simulink model "ship_induction_motor_propulsion_extended_linear"  (R2016b)
settings: Solver=VariableStepAuto  StartTime=0.0  StopTime=500  FixedStep=1e-6
values from neighbouring files (symbols this model uses):
  a = -5.4036    [lin_propulsion_params.m]    (also in robust_lin_propulsion_params_zs.m; ship_induction_motor_propulsion_extended_linear.m)
  b = -3.499    [lin_propulsion_params.m]    (also in robust_lin_propulsion_params_zs.m; ship_induction_motor_propulsion_extended_linear.m)
  J_ind = 4.1    [linear_motor_params.m]    (also in robust_linear_motor_params.m = ureal('J_ind',4.1,'Percentage',range); ship_induction_motor_propulsion_extended_linear.m)
  L_ad_ind = L_aq_ind    (= 0.00307086614173)    [linear_motor_params.m]    (also in robust_linear_motor_params.m = L_aq_ind; ship_induction_motor_propulsion_extended_linear.m)
  L_aq_ind = 1/(1/L_M_ind + 1/L_ls_ind + 1/L_lr_ind)    (= 0.00307086614173)    [linear_motor_params.m]    (also in robust_linear_motor_params.m = 1/(1/L_M_ind + 1/L_ls_ind + 1/L_lr_ind); ship_induction_motor_propulsion_extended_linear.m)
  L_eq = L_ls_ind + L_M_ind *(L_lr_ind)/(L_lr_ind+L_M_ind)    (= 0.0188613861386)    [linear_motor_params.m]    (also in robust_linear_motor_params.m = L_ls_ind + L_M_ind *(L_lr_ind)/(L_lr_ind+L_M_ind); ship_induction_motor_propulsion_extended_linear.m)
  L_lr_ind = 15e-3    (= 0.015)    [linear_motor_params.m]    (also in robust_linear_motor_params.m = ureal('L_lr_ind',15e-3, 'Percentage',range); ship_induction_motor_propulsion_extended_linear.m)
  L_ls_ind = 15e-3    (= 0.015)    [linear_motor_params.m]    (also in robust_linear_motor_params.m = ureal('L_ls_ind',15e-3, 'Percentage',range); ship_induction_motor_propulsion_extended_linear.m)
  L_M_ind = 5.2e-3    (= 0.0052)    [linear_motor_params.m]    (also in robust_linear_motor_params.m = ureal('L_M_ind',5.2e-3, 'Percentage',range); ship_induction_motor_propulsion_extended_linear.m)
  p = 6.58    [lin_propulsion_params.m]    (also in robust_lin_propulsion_params_zs.m; ship_induction_motor_propulsion_extended_linear.m)
  P_ind = 4    [linear_motor_params.m]    (also in robust_linear_motor_params.m; ship_induction_motor_propulsion_extended_linear.m)
  q = 5.0245    [lin_propulsion_params.m]    (also in robust_lin_propulsion_params_zs.m; ship_induction_motor_propulsion_extended_linear.m)
  r_r_ind = 4.6e-3    (= 0.0046)    [linear_motor_params.m]    (also in robust_linear_motor_params.m = ureal('r_r_ind', 4.6e-3, 'Percentage', range); ship_induction_motor_propulsion_extended_linear.m)
  r_s_ind = 7.6e-3    (= 0.0076)    [linear_motor_params.m]    (also in robust_linear_motor_params.m = ureal('r_s_ind', 7.6e-3, 'Percentage', range); ship_induction_motor_propulsion_extended_linear.m)
  T_r_ind = L_lr_ind/r_r_ind    (= 3.26086956522)    [linear_motor_params.m]    (also in robust_linear_motor_params.m = L_lr_ind/r_r_ind; ship_induction_motor_propulsion_extended_linear.m)
  T_s_est = 1e-2    (= 0.01)    [linear_motor_params.m]    (also in robust_linear_motor_params.m; ship_induction_motor_propulsion_extended_linear.m)
  Tn = 7.83    [lin_propulsion_params.m]    (also in robust_lin_propulsion_params_zs.m; ship_induction_motor_propulsion_extended_linear.m)
  Ts = 1e-3    (= 0.001)    [linear_motor_params.m]    (also in robust_linear_motor_params.m; ship_induction_motor_propulsion_extended_linear.m)
  Tth = 2    [lin_propulsion_params.m]    (also in robust_lin_propulsion_params_zs.m; ship_induction_motor_propulsion_extended_linear.m)
  Tv = 115.69    [lin_propulsion_params.m]    (also in robust_lin_propulsion_params_zs.m; ship_induction_motor_propulsion_extended_linear.m)
libraries: simulink x10
settings Model: Creator=z003vh9b  LastModifiedBy=z003vh9b

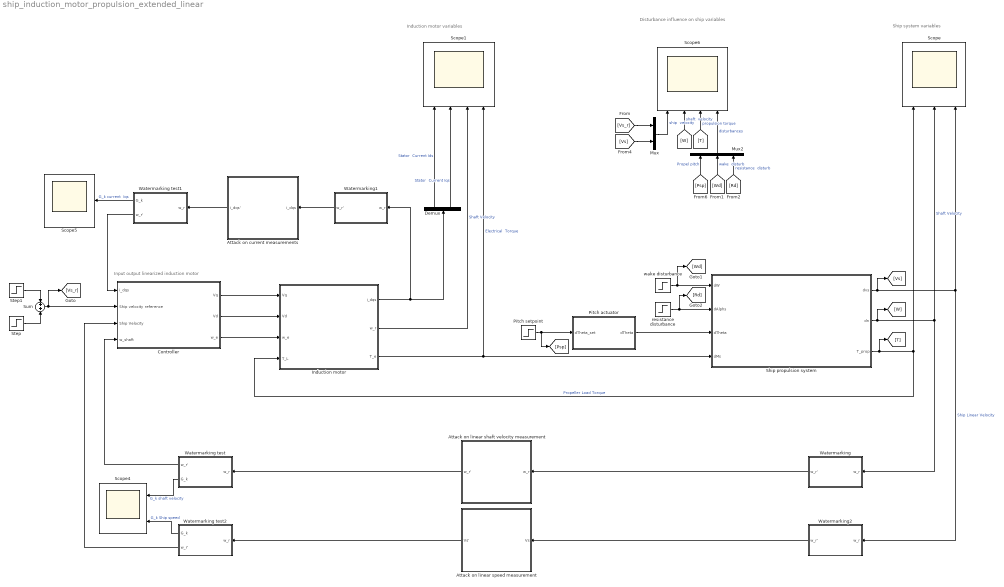
== system ship_induction_motor_propulsion_extended_linear ==
  note: Input output linearized induction motor
  note: Induction motor variables
  note: Ship system variables
  note: Disturbance influence on
      | ship variables
  Attack on current measurements : Subsystem
  Attack on linear shaft velocity measurement : Subsystem
  Attack on linear speed measurement : Subsystem
  Controller : Subsystem
  Demux : Demux  Outputs=2
  Induction motor : Subsystem  mask{N=10e-3, Fs_n=1e3}
      mask prompts: N "Current Noise magnitude"; Fs_n "Current Noise frequency"
  Mux : Mux  Inputs=2
  Mux2 : Mux  Inputs=3
  Pitch actuator : Subsystem
  Pitch setpoint : Step  Time=400  After=-0.5  SampleTime=0
  Scope : Scope  NumInputPorts=3
  Scope1 : Scope  NumInputPorts=4
  Scope4 : Scope  NumInputPorts=2
  Scope5 : Scope
  Scope6 : Scope  NumInputPorts=4
  Ship propulsion system : Subsystem
  Step : Step  Time=200  After=0.5  SampleTime=0
  Step1 : Step  Time=50  SampleTime=0
  Sum : Sum
  Watermarking : Subsystem  mask{N=10e-3, F=1e3, Seed=2}
      mask prompts: N "Noise Magnitude"; F "Noise Frequency"; Seed "Noise Seed"
  Watermarking test : Subsystem  mask{N=10e-3, F=1e3, Seed=2}
      mask prompts: N "Noise Magnitude"; F "Noise Frequency"; Seed "Noise Seed"
  Watermarking test1 : Subsystem  mask{N=20e-3, F=1e3, Seed=4}
      mask prompts: N "Noise Magnitude"; F "Noise Frequency"; Seed "Noise Seed"
  Watermarking test2 : Subsystem  mask{N=10e-3, F=1e3, Seed=3}
      mask prompts: N "Noise Magnitude"; F "Noise Frequency"; Seed "Noise Seed"
  Watermarking1 : Subsystem  mask{N=20e-3, F=1e3, Seed=4}
      mask prompts: N "Noise Magnitude"; F "Noise Frequency"; Seed "Noise Seed"
  Watermarking2 : Subsystem  mask{N=10e-3, F=1e3, Seed=3}
      mask prompts: N "Noise Magnitude"; F "Noise Frequency"; Seed "Noise Seed"
  resistance disturbance : Step  Time=300  After=-0.5  SampleTime=0
  wake disturbance : Step  Time=150  After=-0.5  SampleTime=0
  wires:
  Pitch actuator/1(dTheta) -> Ship propulsion system/3(dTheta)
  Pitch setpoint/1 -> Pitch actuator/1(dTheta_set), [Psp]
  resistance disturbance/1 -> [Rd], Ship propulsion system/2(dAlphs)
  wake disturbance/1 -> [Wd], Ship propulsion system/1(dW)
  Ship propulsion system/1(dvs) -> [Vs], Scope/3, Watermarking2/1(w_r)  "Ship Linear Velocity"
  Ship propulsion system/2(dn) -> [W], Watermarking/1(w_r), Scope/2  "Shaft Velocity"
  Ship propulsion system/3(T_prop) -> [T], Induction motor/4(T_L), Scope/1  "Propeller Load Torque"
  Induction motor/2(w_r) -> Scope1/3  "Shaft Velocity"
  Induction motor/3(T_e) -> Ship propulsion system/4(dMs), Scope1/4  "Electrical  Torque"
  Sum/1 -> Controller/2(Ship velocity reference), [Vs_r]
  Controller/1(Vq) -> Induction motor/1(Vq)
  Controller/2(Vd) -> Induction motor/2(Vd)
  Controller/3(w_e) -> Induction motor/3(w_e)
  Demux/1 -> Scope1/1  "Stator  Current Ids"
  Demux/2 -> Scope1/2  "Stator  Current Iqs"
  Watermarking test/1(w_r') -> Controller/4(w_shaft)
  Watermarking/1(w_r') -> Attack on linear shaft velocity measurement/1(w_r)
  Watermarking2/1(w_r') -> Attack on linear speed measurement/1(Vs)
  Watermarking test/2(G_k) -> Scope4/1  "G_k shaft velocity"
  Attack on linear speed measurement/1(Vs') -> Watermarking test2/1(w_r)
  Watermarking test2/1(G_k) -> Scope4/2  "G_k Ship speed"
  Attack on linear shaft velocity measurement/1(w_r') -> Watermarking test/1(w_r)
  Watermarking test2/2(w_r') -> Controller/3(Ship Velocity)
  Induction motor/1(i_dqs) -> Demux/1, Watermarking1/1(w_r)
  Attack on current measurements/1(i_dqs') -> Watermarking test1/1(w_r)
  Watermarking test1/1(G_k) -> Scope5/1  "G_k current  Iqs"
  Step/1 -> Sum/2
  Step1/1 -> Sum/1
  Watermarking1/1(w_r') -> Attack on current measurements/1(i_dqs)
  Watermarking test1/2(w_r') -> Controller/1(i_dqs)
  [Wd] -> Mux2/2  "wake  disturb"
  [Rd] -> Mux2/3  "resistance  disturb"
  [Vs_r] -> Mux/1
  [Vs] -> Mux/2
  Mux/1 -> Scope6/1  "ship  velocity"
  Mux2/1 -> Scope6/4  "disturbances"
  [W] -> Scope6/2  "shaft  velocity"
  [Psp] -> Mux2/1  "Propel pitch"
  [T] -> Scope6/3  "propulsion torque"

== system ship_induction_motor_propulsion_extended_linear/Attack on current measurements ==
  i_dqs : Inport
  Demux : Demux  Outputs=2
  Mux : Mux  Inputs=2
  Repeating Sequence Stair : simulink/Sources/Repeating Sequence Stair  OutValues=[0 11].'  tsamp=80  OutMin=[]  OutMax=[]  OutDataTypeStr=double  OutputDataTypeScalingMode=double  OutDataType=fixdt(0,8)  ConRadixGroup=Best Precision: Vector-wise  OutScaling=2^-12
  Variable Integer Delay : Delay  DelayLengthSource=Input port  SampleTime=Ts
      settings: InputPortMap=u0,p1
  i_dqs' : Outport
  wires:
  Mux/1 -> i_dqs'/1
  i_dqs/1 -> Demux/1
  Demux/1 -> Mux/1
  Variable Integer Delay/1 -> Mux/2
  Demux/2 -> Variable Integer Delay/1
  Repeating Sequence Stair/1 -> Variable Integer Delay/2

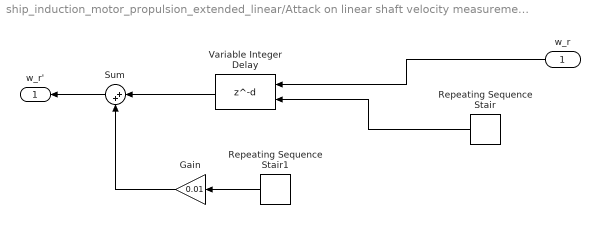
== system ship_induction_motor_propulsion_extended_linear/Attack on linear shaft velocity measurement ==
  w_r : Inport
  Gain : Gain  Gain=0.01
  Repeating Sequence Stair : simulink/Sources/Repeating Sequence Stair  OutValues=[0 3000 5 0 0].'  tsamp=80  OutMin=[]  OutMax=[]  OutDataTypeStr=double  OutputDataTypeScalingMode=double  OutDataType=fixdt(0,8)  ConRadixGroup=Best Precision: Vector-wise  OutScaling=2^-12
  Repeating Sequence Stair1 : simulink/Sources/Repeating Sequence Stair  OutValues="[0 0 0 0  1].'"  tsamp=80  OutMin=[]  OutMax=[]  OutDataTypeStr=double  OutputDataTypeScalingMode=double  OutDataType=fixdt(0,8)  ConRadixGroup=Best Precision: Vector-wise  OutScaling=2^-12
  Sum : Sum  Inputs=|++
  Variable Integer Delay : Delay  DelayLengthSource=Input port  SampleTime=Ts
      settings: InputPortMap=u0,p1
  w_r' : Outport
  wires:
  Variable Integer Delay/1 -> Sum/1
  w_r/1 -> Variable Integer Delay/1
  Repeating Sequence Stair/1 -> Variable Integer Delay/2
  Sum/1 -> w_r'/1
  Repeating Sequence Stair1/1 -> Gain/1
  Gain/1 -> Sum/2

== system ship_induction_motor_propulsion_extended_linear/Attack on linear speed measurement ==
  Vs : Inport
  Repeating Sequence Stair : simulink/Sources/Repeating Sequence Stair  OutValues=[0 1 2 3 0].'  tsamp=80  OutMin=[]  OutMax=[]  OutDataTypeStr=double  OutputDataTypeScalingMode=double  OutDataType=fixdt(0,8)  ConRadixGroup=Best Precision: Vector-wise  OutScaling=2^-12
  Variable Integer Delay : Delay  DelayLengthSource=Input port  SampleTime=Ts
      settings: InputPortMap=u0,p1
  Vs' : Outport
  wires:
  Variable Integer Delay/1 -> Vs'/1
  Vs/1 -> Variable Integer Delay/1
  Repeating Sequence Stair/1 -> Variable Integer Delay/2

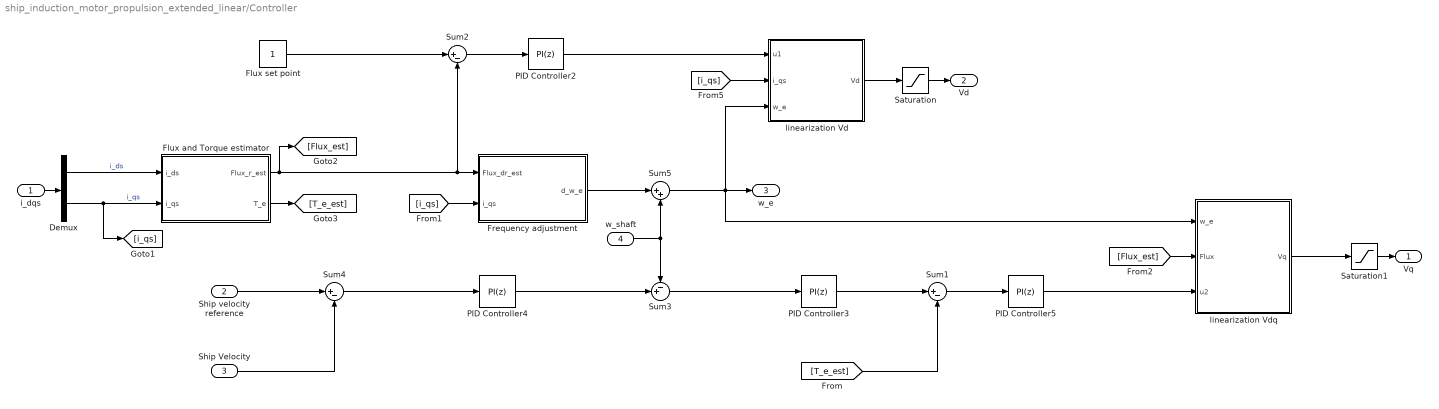
== system ship_induction_motor_propulsion_extended_linear/Controller ==
  i_dqs : Inport
  Ship velocity reference : Inport  Port=2
  Ship Velocity : Inport  Port=3
  w_shaft : Inport  Port=4
  Demux : Demux  Outputs=2
  Flux and Torque estimator : Subsystem
  Flux set point : Constant
  Frequency adjustment : Subsystem
  PID Controller2 : simulink/Continuous/PID Controller  Controller=PI  TimeDomain=Discrete-time  SampleTime=0.01  IntegratorMethod=Forward Euler  FilterMethod=Forward Euler  Form=Parallel  UseFilter=on  ControllerParametersSource=internal  P=1  I=0.1  D=0  N=100  InitialConditionSource=internal  InitialConditionForIntegrator=0  InitialConditionForFilter=0  ExternalReset=none  LimitOutput=off  UpperSaturationLimit=inf  LowerSaturationLimit=-inf  LinearizeAsGain=on  AntiWindupMode=none  Kb=1  TrackingMode=off  Kt=1  PParamMin=[]  PParamMax=[]  IParamMin=[]  IParamMax=[]  DParamMin=[]  DParamMax=[]  NParamMin=[]  NParamMax=[]  KbParamMin=[]  KbParamMax=[]  KtParamMin=[]  KtParamMax=[]  POutMin=[]  POutMax=[]  IOutMin=[]  IOutMax=[]  DOutMin=[]  DOutMax=[]  NOutMin=[]  NOutMax=[]  KbOutMin=[]  KbOutMax=[]  KtOutMin=[]  KtOutMax=[]  IntegratorOutMin=[]  IntegratorOutMax=[]  FilterOutMin=[]  FilterOutMax=[]  SumOutMin=[]  SumOutMax=[]  SumI1OutMin=[]  SumI1OutMax=[]  SumI2OutMin=[]  SumI2OutMax=[]  SumI3OutMin=[]  SumI3OutMax=[]  SumDOutMin=[]  SumDOutMax=[]  SaturationOutMin=[]  SaturationOutMax=[]  IntegratorContinuousStateAttributes=''  IntegratorStateMustResolveToSignalObject=off  IntegratorRTWStateStorageClass=Auto  FilterContinuousStateAttributes=''  FilterStateMustResolveToSignalObject=off  FilterRTWStateStorageClass=Auto  DifferentiatorICPrevScaledInput=0  DifferentiatorOutMin=[]  DifferentiatorOutMax=[]
  PID Controller3 : simulink/Continuous/PID Controller  Controller=PI  TimeDomain=Discrete-time  SampleTime=Ts  IntegratorMethod=Forward Euler  FilterMethod=Forward Euler  Form=Parallel  UseFilter=on  ControllerParametersSource=internal  P=10  I=10  D=1  N=100  InitialConditionSource=internal  InitialConditionForIntegrator=0  InitialConditionForFilter=0  ExternalReset=none  LimitOutput=off  UpperSaturationLimit=inf  LowerSaturationLimit=-inf  LinearizeAsGain=on  AntiWindupMode=none  Kb=1  TrackingMode=off  Kt=1  PParamMin=[]  PParamMax=[]  IParamMin=[]  IParamMax=[]  DParamMin=[]  DParamMax=[]  NParamMin=[]  NParamMax=[]  KbParamMin=[]  KbParamMax=[]  KtParamMin=[]  KtParamMax=[]  POutMin=[]  POutMax=[]  IOutMin=[]  IOutMax=[]  DOutMin=[]  DOutMax=[]  NOutMin=[]  NOutMax=[]  KbOutMin=[]  KbOutMax=[]  KtOutMin=[]  KtOutMax=[]  IntegratorOutMin=[]  IntegratorOutMax=[]  FilterOutMin=[]  FilterOutMax=[]  SumOutMin=[]  SumOutMax=[]  SumI1OutMin=[]  SumI1OutMax=[]  SumI2OutMin=[]  SumI2OutMax=[]  SumI3OutMin=[]  SumI3OutMax=[]  SumDOutMin=[]  SumDOutMax=[]  SaturationOutMin=[]  SaturationOutMax=[]  IntegratorContinuousStateAttributes=''  IntegratorStateMustResolveToSignalObject=off  IntegratorRTWStateStorageClass=Auto  FilterContinuousStateAttributes=''  FilterStateMustResolveToSignalObject=off  FilterRTWStateStorageClass=Auto  DifferentiatorICPrevScaledInput=0  DifferentiatorOutMin=[]  DifferentiatorOutMax=[]
  PID Controller4 : simulink/Continuous/PID Controller  Controller=PI  TimeDomain=Discrete-time  SampleTime=Ts  IntegratorMethod=Forward Euler  FilterMethod=Forward Euler  Form=Parallel  UseFilter=on  ControllerParametersSource=internal  P=1  I=0.1  D=1  N=100  InitialConditionSource=internal  InitialConditionForIntegrator=0  InitialConditionForFilter=0  ExternalReset=none  LimitOutput=off  UpperSaturationLimit=inf  LowerSaturationLimit=-inf  LinearizeAsGain=on  AntiWindupMode=none  Kb=1  TrackingMode=off  Kt=1  PParamMin=[]  PParamMax=[]  IParamMin=[]  IParamMax=[]  DParamMin=[]  DParamMax=[]  NParamMin=[]  NParamMax=[]  KbParamMin=[]  KbParamMax=[]  KtParamMin=[]  KtParamMax=[]  POutMin=[]  POutMax=[]  IOutMin=[]  IOutMax=[]  DOutMin=[]  DOutMax=[]  NOutMin=[]  NOutMax=[]  KbOutMin=[]  KbOutMax=[]  KtOutMin=[]  KtOutMax=[]  IntegratorOutMin=[]  IntegratorOutMax=[]  FilterOutMin=[]  FilterOutMax=[]  SumOutMin=[]  SumOutMax=[]  SumI1OutMin=[]  SumI1OutMax=[]  SumI2OutMin=[]  SumI2OutMax=[]  SumI3OutMin=[]  SumI3OutMax=[]  SumDOutMin=[]  SumDOutMax=[]  SaturationOutMin=[]  SaturationOutMax=[]  IntegratorContinuousStateAttributes=''  IntegratorStateMustResolveToSignalObject=off  IntegratorRTWStateStorageClass=Auto  FilterContinuousStateAttributes=''  FilterStateMustResolveToSignalObject=off  FilterRTWStateStorageClass=Auto  DifferentiatorICPrevScaledInput=0  DifferentiatorOutMin=[]  DifferentiatorOutMax=[]
  PID Controller5 : simulink/Continuous/PID Controller  Controller=PI  TimeDomain=Discrete-time  SampleTime=Ts  IntegratorMethod=Forward Euler  FilterMethod=Forward Euler  Form=Parallel  UseFilter=on  ControllerParametersSource=internal  P=1  I=10  D=1  N=100  InitialConditionSource=internal  InitialConditionForIntegrator=0  InitialConditionForFilter=0  ExternalReset=none  LimitOutput=off  UpperSaturationLimit=500  LowerSaturationLimit=-500  LinearizeAsGain=on  AntiWindupMode=none  Kb=1  TrackingMode=off  Kt=1  PParamMin=[]  PParamMax=[]  IParamMin=[]  IParamMax=[]  DParamMin=[]  DParamMax=[]  NParamMin=[]  NParamMax=[]  KbParamMin=[]  KbParamMax=[]  KtParamMin=[]  KtParamMax=[]  POutMin=[]  POutMax=[]  IOutMin=[]  IOutMax=[]  DOutMin=[]  DOutMax=[]  NOutMin=[]  NOutMax=[]  KbOutMin=[]  KbOutMax=[]  KtOutMin=[]  KtOutMax=[]  IntegratorOutMin=[]  IntegratorOutMax=[]  FilterOutMin=[]  FilterOutMax=[]  SumOutMin=[]  SumOutMax=[]  SumI1OutMin=[]  SumI1OutMax=[]  SumI2OutMin=[]  SumI2OutMax=[]  SumI3OutMin=[]  SumI3OutMax=[]  SumDOutMin=[]  SumDOutMax=[]  SaturationOutMin=[]  SaturationOutMax=[]  IntegratorContinuousStateAttributes=''  IntegratorStateMustResolveToSignalObject=off  IntegratorRTWStateStorageClass=Auto  FilterContinuousStateAttributes=''  FilterStateMustResolveToSignalObject=off  FilterRTWStateStorageClass=Auto  DifferentiatorICPrevScaledInput=0  DifferentiatorOutMin=[]  DifferentiatorOutMax=[]
  Saturation : Saturate  UpperLimit=100  LowerLimit=-100
  Saturation1 : Saturate  UpperLimit=100  LowerLimit=-100
  Sum1 : Sum  Inputs=|+-
  Sum2 : Sum  Inputs=|+-
  Sum3 : Sum  Inputs=-+|
  Sum4 : Sum  Inputs=|+-
  Sum5 : Sum  Inputs=|++
  linearization Vd : Subsystem
  linearization Vdq : Subsystem
  Vq : Outport
  Vd : Outport  Port=2
  w_e : Outport  Port=3
  wires:
  PID Controller2/1 -> linearization Vd/1(u1)
  Sum2/1 -> PID Controller2/1
  Sum5/1 -> w_e/1, linearization Vdq/1(w_e), linearization Vd/3(w_e)
  Flux and Torque estimator/1(Flux_r_est) -> Frequency adjustment/1(Flux_dr_est), Sum2/2, [Flux_est]
  w_shaft/1 -> Sum3/1, Sum5/2
  Ship Velocity/1 -> Sum4/2
  Frequency adjustment/1(d_w_e) -> Sum5/1
  Flux set point/1 -> Sum2/1
  Ship velocity reference/1 -> Sum4/1
  PID Controller4/1 -> Sum3/2
  Sum3/1 -> PID Controller3/1
  Sum4/1 -> PID Controller4/1
  [i_qs] -> Frequency adjustment/2(i_qs)
  Demux/1 -> Flux and Torque estimator/1(i_ds)  "i_ds"
  Demux/2 -> Flux and Torque estimator/2(i_qs), [i_qs]  "i_qs"
  i_dqs/1 -> Demux/1
  [i_qs] -> linearization Vd/2(i_qs)
  Sum1/1 -> PID Controller5/1
  Flux and Torque estimator/2(T_e) -> [T_e_est]
  [Flux_est] -> linearization Vdq/2(Flux)
  linearization Vd/1(Vd) -> Saturation/1
  linearization Vdq/1(Vq) -> Saturation1/1
  PID Controller3/1 -> Sum1/1
  [T_e_est] -> Sum1/2
  PID Controller5/1 -> linearization Vdq/3(u2)
  Saturation/1 -> Vd/1
  Saturation1/1 -> Vq/1

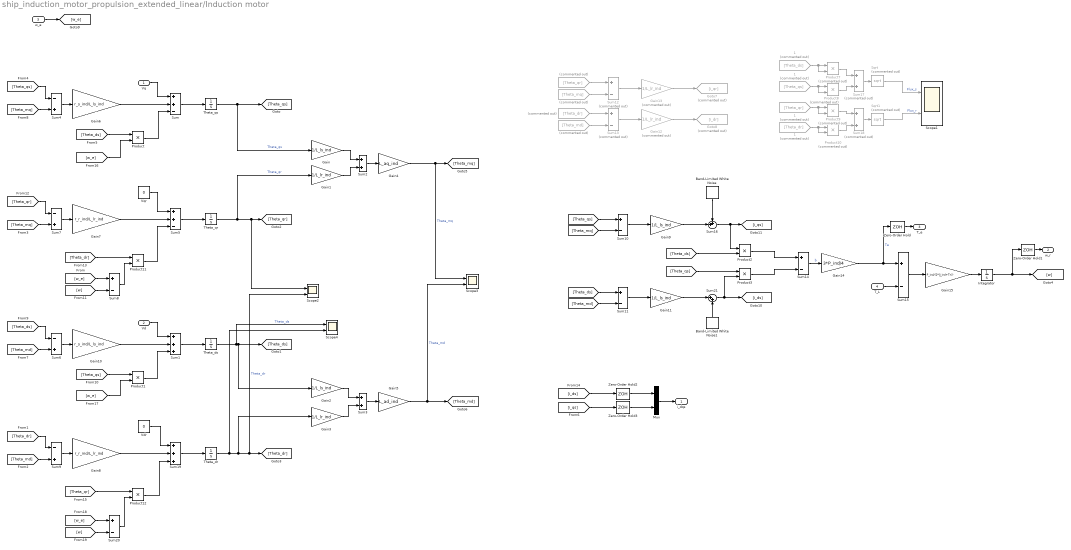
== system ship_induction_motor_propulsion_extended_linear/Induction motor ==
  Vq : Inport
  Vd : Inport  Port=2
  w_e : Inport  Port=3
  T_L : Inport  Port=4
  "    " : From  Commented=on  GotoTag=Theta_dr
  "         " : From  Commented=on  GotoTag=Theta_md
  "          " : From  Commented=on  GotoTag=Theta_qr
  "            " : From  Commented=on  GotoTag=Theta_mq
  "          1" : From  Commented=on  GotoTag=Theta_qr
  "    1" : From  Commented=on  GotoTag=Theta_dr
  "   1" : From  Commented=on  GotoTag=Theta_qs
  " 1" : From  Commented=on  GotoTag=Theta_ds
  Band-Limited White Noise : simulink/Sources/Band-Limited White Noise  Cov=N^2/( Fs_n*2*pi)  Ts=1/Fs_n  seed=[2331]
  Band-Limited White Noise1 : simulink/Sources/Band-Limited White Noise  Cov=N^2/( Fs_n*2*pi)  Ts=1/Fs_n  seed=[2343231]
  Gain{,2,9,11} (4 alike) : Gain  Gain=1/L_ls_ind
  Gain1 : Gain  Gain=1/L_lr_ind
  Gain10 : Gain  Gain=r_s_ind/L_ls_ind
  Gain12 : Gain  Commented=on  Gain=1/L_lr_ind
  Gain13 : Gain  Commented=on  Gain=1/L_lr_ind
  Gain14 : Gain  Gain=3*P_ind/4
  Gain15 : Gain  Gain=P_ind/(2*(J_ind+Tn))
  Gain3 : Gain  Gain=1/L_lr_ind
  Gain4 : Gain  Gain=L_aq_ind
  Gain5 : Gain  Gain=L_ad_ind
  Gain6 : Gain  Gain=r_s_ind/L_ls_ind
  Gain7 : Gain  Gain=r_r_ind/L_lr_ind
  Gain8 : Gain  Gain=r_r_ind/L_lr_ind
  Goto7 : Goto  Commented=on  GotoTag=i_qr
  Goto8 : Goto  Commented=on  GotoTag=i_dr
  Integrator : Integrator
  Mux : Mux  Inputs=2
  Product{,1..3,11..12} (6 alike) : Product
  Product{7..10} (4 alike) : Product  Commented=on
  Scope{1..4} (4 alike) : Scope  NumInputPorts=2
  Sqrt : Sqrt  Commented=on  SaturateOnIntegerOverflow=on
  Sqrt1 : Sqrt  Commented=on  SaturateOnIntegerOverflow=on
  Sum : Sum  Inputs=++-
  Sum1 : Sum  Inputs=+++
  Sum{8,10..11,14..15,20} (6 alike) : Sum  Inputs=+-
  Sum12 : Sum  Commented=on  Inputs=+-
  Sum13 : Sum  Commented=on  Inputs=+-
  Sum16 : Sum  Inputs=++|
  Sum17 : Sum  Commented=on
  Sum18 : Sum  Commented=on
  Sum19 : Sum  Inputs=+++
  Sum2 : Sum
  Sum21 : Sum  Inputs=|++
  Sum3 : Sum
  Sum{4,6..7,9} (4 alike) : Sum  Inputs=-+
  Sum5 : Sum  Inputs=++-
  Theta_dr : Integrator  InitialCondition=1
  Theta_ds : Integrator  InitialCondition=4
  Theta_qr : Integrator
  Theta_qs : Integrator
  Vdr : Constant  Value=0
  Vqr : Constant  Value=0
  Zero-Order Hold{,1..3} (4 alike) : ZeroOrderHold  SampleTime=Ts
  i_dqs : Outport
  w_r : Outport  Port=2
  T_e : Outport  Port=3
  wires:
  Vq/1 -> Sum/1
  Vd/1 -> Sum1/1
  Sum1/1 -> Theta_ds/1
  Sum/1 -> Theta_qs/1
  Theta_qs/1 -> [Theta_qs], Gain/1  "Theta_qs"
  Theta_ds/1 -> Scope4/1, [Theta_ds], Gain2/1  "Theta_ds"
  Theta_qr/1 -> Gain1/1, Scope2/1, [Theta_qr]  "Theta_qr"
  Theta_dr/1 -> Scope4/2, Scope2/2, [Theta_dr], Gain3/1  "Theta_dr"
  [Theta_qs] -> Sum4/1
  Sum4/1 -> Gain6/1
  Gain6/1 -> Sum/2
  [Theta_ds] -> Product/1
  Product/1 -> Sum/3
  [w_e] -> Product/2
  [Theta_ds] -> Sum6/1
  Sum6/1 -> Gain10/1
  Gain10/1 -> Sum1/2
  [Theta_qs] -> Product1/1
  [w_e] -> Product1/2
  Product1/1 -> Sum1/3
  Gain/1 -> Sum2/1
  Gain1/1 -> Sum2/2
  Sum2/1 -> Gain4/1
  Gain4/1 -> Scope3/1, [Theta_mq]  "Theta_mq"
  Gain2/1 -> Sum3/1
  Gain3/1 -> Sum3/2
  Sum3/1 -> Gain5/1
  Gain5/1 -> Scope3/2, [Theta_md]  "Theta_md"
  [Theta_mq] -> Sum4/2
  [Theta_md] -> Sum6/2
  Vqr/1 -> Sum5/1
  Sum5/1 -> Theta_qr/1
  [Theta_qr] -> Sum7/1
  Sum7/1 -> Gain7/1
  Gain7/1 -> Sum5/2
  [Theta_mq] -> Sum7/2
  Vdr/1 -> Sum19/1
  Sum19/1 -> Theta_dr/1
  [Theta_dr] -> Sum9/1
  Sum9/1 -> Gain8/1
  Gain8/1 -> Sum19/2
  [Theta_md] -> Sum9/2
  Sum16/1 -> [i_qs], Product2/1
  Sum21/1 -> Product3/2, [i_ds]
  Sum12/1 -> Gain13/1
  Sum13/1 -> Gain12/1
  [Theta_qs] -> Sum10/1
  [Theta_mq] -> Sum10/2
  "          "/1 -> Sum12/1
  "            "/1 -> Sum12/2
  "    "/1 -> Sum13/1
  "         "/1 -> Sum13/2
  [Theta_qs] -> Product3/1
  [Theta_ds] -> Product2/2
  Product2/1 -> Sum14/1
  Product3/1 -> Sum14/2
  Sum14/1 -> Gain14/1  "b"
  Gain14/1 -> Zero-Order Hold/1, Sum15/1  "Te"
  T_L/1 -> Sum15/2
  Sum15/1 -> Gain15/1
  Gain15/1 -> Integrator/1
  Integrator/1 -> Zero-Order Hold1/1, [w]
  Sum10/1 -> Gain9/1
  [Theta_ds] -> Sum11/1
  [Theta_md] -> Sum11/2
  Sum11/1 -> Gain11/1
  Gain13/1 -> Goto7/1
  Gain12/1 -> Goto8/1
  Sqrt/1 -> Scope1/1  "Flux_s"
  Sqrt1/1 -> Scope1/2  "Flux_r"
  Sum17/1 -> Sqrt/1
  Sum18/1 -> Sqrt1/1
  Product9/1 -> Sum18/1
  Product10/1 -> Sum18/2
  Product8/1 -> Sum17/2
  Product7/1 -> Sum17/1
  "    1"/1 -> Product10/2, Product10/1
  "          1"/1 -> Product9/1, Product9/2
  "   1"/1 -> Product8/2, Product8/1
  " 1"/1 -> Product7/2, Product7/1
  [Theta_dr] -> Product11/1
  Product11/1 -> Sum5/3
  [w_e] -> Sum8/1
  [Theta_qr] -> Product12/1
  Product12/1 -> Sum19/3
  w_e/1 -> [w_e]
  [w] -> Sum8/2
  Sum8/1 -> Product11/2
  [w_e] -> Sum20/1
  [w] -> Sum20/2
  Sum20/1 -> Product12/2
  Mux/1 -> i_dqs/1
  Band-Limited White Noise/1 -> Sum16/1
  Gain9/1 -> Sum16/2
  Band-Limited White Noise1/1 -> Sum21/2
  Gain11/1 -> Sum21/1
  Zero-Order Hold/1 -> T_e/1
  Zero-Order Hold1/1 -> w_r/1
  [i_ds] -> Zero-Order Hold2/1
  [i_qs] -> Zero-Order Hold3/1
  Zero-Order Hold2/1 -> Mux/1
  Zero-Order Hold3/1 -> Mux/2

== system ship_induction_motor_propulsion_extended_linear/Pitch actuator ==
  dTheta_set : Inport
  Transfer Fcn : TransferFcn  Denominator=[Tth 1]
  dTheta : Outport
  wires:
  dTheta_set/1 -> Transfer Fcn/1
  Transfer Fcn/1 -> dTheta/1

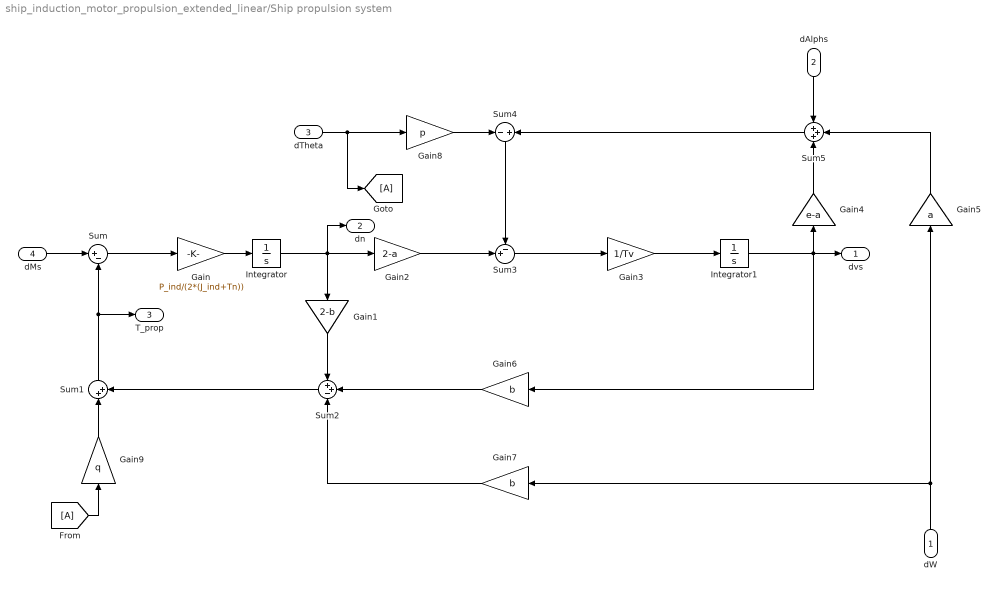
== system ship_induction_motor_propulsion_extended_linear/Ship propulsion system ==
  dW : Inport
  dAlphs : Inport  Port=2
  dTheta : Inport  Port=3
  dMs : Inport  Port=4
  Gain : Gain  Gain=P_ind/(2*(J_ind+Tn))
  Gain1 : Gain  Gain=2-b
  Gain2 : Gain  Gain=2-a
  Gain3 : Gain  Gain=1/Tv
  Gain4 : Gain  Gain=e-a
  Gain5 : Gain  Gain=a
  Gain6 : Gain  Gain=b
  Gain7 : Gain  Gain=b
  Gain8 : Gain  Gain=p
  Gain9 : Gain  Gain=q
  Integrator : Integrator
  Integrator1 : Integrator
  Sum : Sum  Inputs=|+-
  Sum1 : Sum  Inputs=|++
  Sum2 : Sum  Inputs=++-
  Sum3 : Sum  Inputs=-+|
  Sum4 : Sum  Inputs=-+
  Sum5 : Sum  Inputs=+++
  dvs : Outport
  dn : Outport  Port=2
  T_prop : Outport  Port=3
  wires:
  Sum1/1 -> T_prop/1, Sum/2
  Sum/1 -> Gain/1
  Gain/1 -> Integrator/1
  Integrator/1 -> dn/1, Gain1/1, Gain2/1
  Gain2/1 -> Sum3/2
  Sum4/1 -> Sum3/1
  Sum3/1 -> Gain3/1
  Gain8/1 -> Sum4/1
  Sum5/1 -> Sum4/2
  Gain4/1 -> Sum5/3
  Integrator1/1 -> dvs/1, Gain6/1, Gain4/1
  Gain3/1 -> Integrator1/1
  Gain5/1 -> Sum5/2
  Gain7/1 -> Sum2/3
  Gain6/1 -> Sum2/2
  Gain1/1 -> Sum2/1
  Sum2/1 -> Sum1/2
  Gain9/1 -> Sum1/1
  dW/1 -> Gain5/1, Gain7/1
  dAlphs/1 -> Sum5/1
  dTheta/1 -> [A], Gain8/1
  [A] -> Gain9/1
  dMs/1 -> Sum/1

== system ship_induction_motor_propulsion_extended_linear/Watermarking ==
  w_r : Inport
  Mux : Mux  Inputs=2
  Noise Generation : MATLAB Function  TreatAsAtomicUnit=on  SystemSampleTime=Ts
  Scope : Scope  NumInputPorts=3
  w_r' : Outport
  wires:
  w_r/1 -> Mux/2, Noise Generation/1(x)
  Noise Generation/3(x_noise) -> Mux/1, w_r'/1
  Mux/1 -> Scope/3
  Noise Generation/2(hashing_noise) -> Scope/2
  Noise Generation/1(prs_noise) -> Scope/1

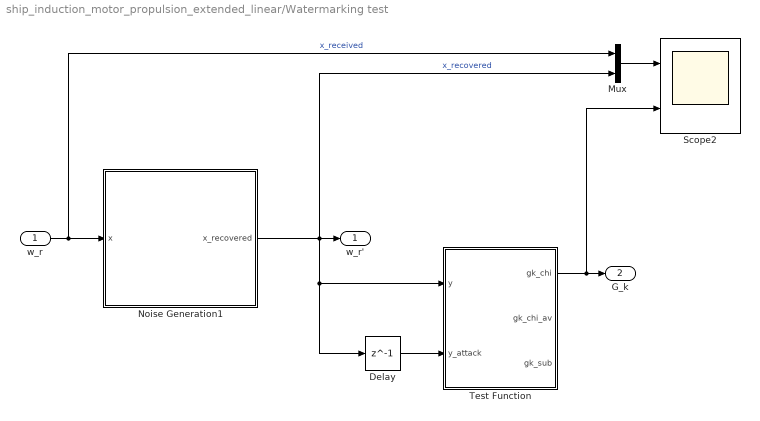
== system ship_induction_motor_propulsion_extended_linear/Watermarking test ==
  w_r : Inport
  Delay : Delay  DelayLength=1  InitialCondition=0  SampleTime=1/F
  Mux : Mux  Inputs=2
  Noise Generation1 : MATLAB Function  TreatAsAtomicUnit=on  SystemSampleTime=1/F
  Scope2 : Scope  NumInputPorts=2
  Test Function : MATLAB Function  TreatAsAtomicUnit=on  SystemSampleTime=1/F
  w_r' : Outport
  G_k : Outport  Port=2
  wires:
  Delay/1 -> Test Function/2(y_attack)
  Noise Generation1/1(x_recovered) -> Mux/2, Delay/1, Test Function/1(y), w_r'/1  "x_recovered"
  Test Function/1(gk_chi) -> Scope2/2, G_k/1
  w_r/1 -> Mux/1, Noise Generation1/1(x)  "x_received"
  Mux/1 -> Scope2/1

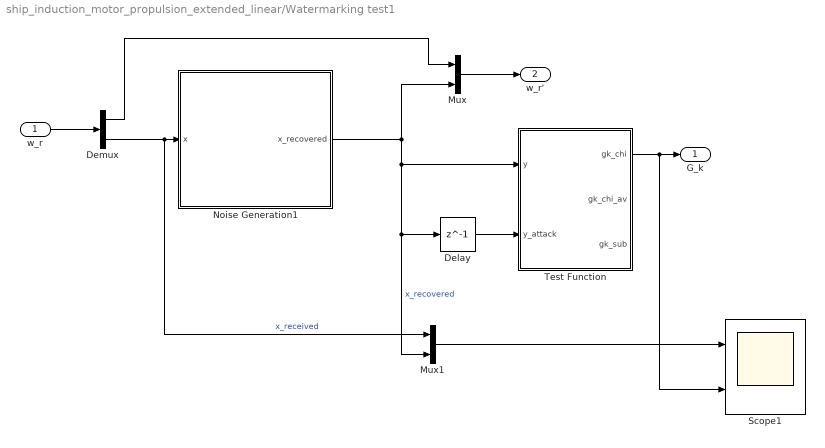
== system ship_induction_motor_propulsion_extended_linear/Watermarking test1 ==
  w_r : Inport
  Delay : Delay  DelayLength=1  InitialCondition=0  SampleTime=1/F
  Demux : Demux  Outputs=2
  Mux : Mux  Inputs=2
  Mux1 : Mux  Inputs=2
  Noise Generation1 : MATLAB Function  TreatAsAtomicUnit=on  SystemSampleTime=1/F
  Scope1 : Scope  NumInputPorts=2
  Test Function : MATLAB Function  TreatAsAtomicUnit=on  SystemSampleTime=1/F
  G_k : Outport
  w_r' : Outport  Port=2
  wires:
  Delay/1 -> Test Function/2(y_attack)
  w_r/1 -> Demux/1
  Mux/1 -> w_r'/1
  Demux/1 -> Mux/1
  Noise Generation1/1(x_recovered) -> Mux1/2, Delay/1, Test Function/1(y), Mux/2  "x_recovered"
  Test Function/1(gk_chi) -> Scope1/2, G_k/1
  Demux/2 -> Mux1/1, Noise Generation1/1(x)  "x_received"
  Mux1/1 -> Scope1/1

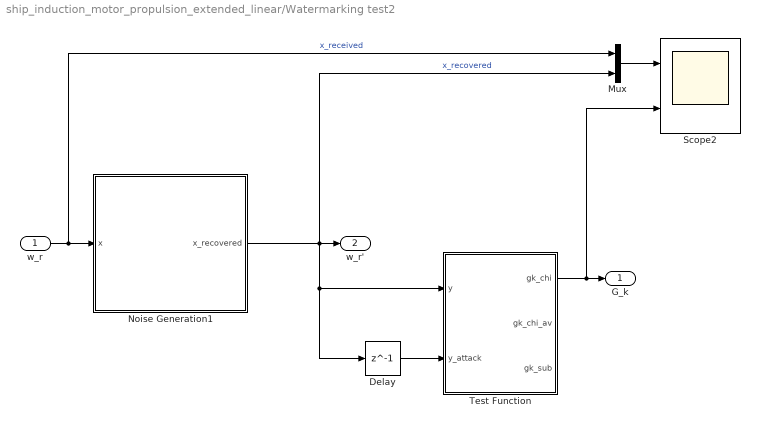
== system ship_induction_motor_propulsion_extended_linear/Watermarking test2 ==
  w_r : Inport
  Delay : Delay  DelayLength=1  InitialCondition=0  SampleTime=1/F
  Mux : Mux  Inputs=2
  Noise Generation1 : MATLAB Function  TreatAsAtomicUnit=on  SystemSampleTime=1/F
  Scope2 : Scope  NumInputPorts=2
  Test Function : MATLAB Function  TreatAsAtomicUnit=on  SystemSampleTime=1/F
  G_k : Outport
  w_r' : Outport  Port=2
  wires:
  Delay/1 -> Test Function/2(y_attack)
  Noise Generation1/1(x_recovered) -> Mux/2, Test Function/1(y), Delay/1, w_r'/1  "x_recovered"
  Test Function/1(gk_chi) -> Scope2/2, G_k/1
  w_r/1 -> Mux/1, Noise Generation1/1(x)  "x_received"
  Mux/1 -> Scope2/1

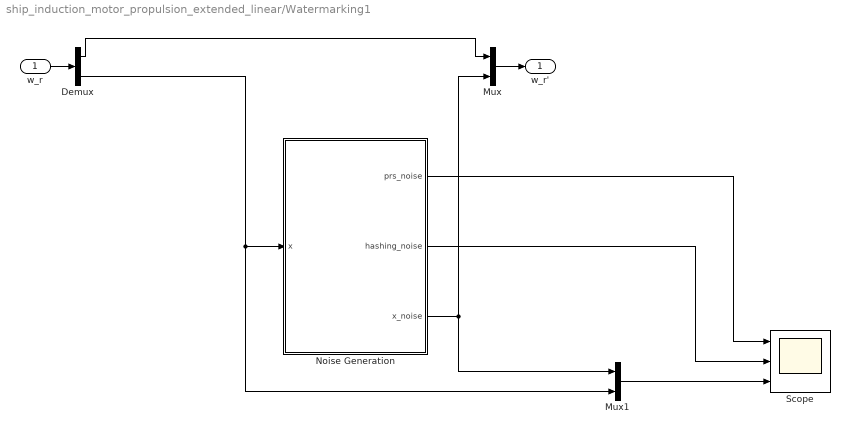
== system ship_induction_motor_propulsion_extended_linear/Watermarking1 ==
  w_r : Inport
  Demux : Demux  Outputs=2
  Mux : Mux  Inputs=2
  Mux1 : Mux  Inputs=2
  Noise Generation : MATLAB Function  TreatAsAtomicUnit=on  SystemSampleTime=Ts
  Scope : Scope  NumInputPorts=3
  w_r' : Outport
  wires:
  w_r/1 -> Demux/1
  Mux/1 -> w_r'/1
  Demux/1 -> Mux/1
  Noise Generation/3(x_noise) -> Mux1/1, Mux/2
  Mux1/1 -> Scope/3
  Noise Generation/2(hashing_noise) -> Scope/2
  Noise Generation/1(prs_noise) -> Scope/1
  Demux/2 -> Mux1/2, Noise Generation/1(x)

== system ship_induction_motor_propulsion_extended_linear/Watermarking2 ==
  w_r : Inport
  Mux : Mux  Inputs=2
  Noise Generation : MATLAB Function  TreatAsAtomicUnit=on  SystemSampleTime=Ts
  Scope : Scope  NumInputPorts=3
  w_r' : Outport
  wires:
  w_r/1 -> Mux/2, Noise Generation/1(x)
  Noise Generation/3(x_noise) -> Mux/1, w_r'/1
  Mux/1 -> Scope/3
  Noise Generation/2(hashing_noise) -> Scope/2
  Noise Generation/1(prs_noise) -> Scope/1

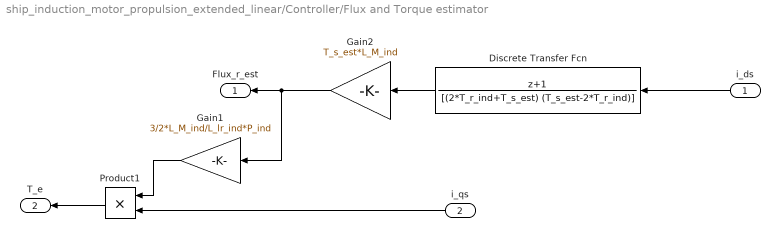
== system ship_induction_motor_propulsion_extended_linear/Controller/Flux and Torque estimator ==
  i_ds : Inport
  i_qs : Inport  Port=2
  Discrete Transfer Fcn : DiscreteTransferFcn  Numerator=[1 1]  Denominator=[(2*T_r_ind+T_s_est) (T_s_est-2*T_r_ind)]  SampleTime=T_s_est
  Gain1 : Gain  Gain=3/2*L_M_ind/L_lr_ind*P_ind
  Gain2 : Gain  Gain=T_s_est*L_M_ind
  Product1 : Product
  Flux_r_est : Outport
  T_e : Outport  Port=2
  wires:
  i_qs/1 -> Product1/2
  Gain2/1 -> Flux_r_est/1, Gain1/1
  Gain1/1 -> Product1/1
  i_ds/1 -> Discrete Transfer Fcn/1
  Product1/1 -> T_e/1
  Discrete Transfer Fcn/1 -> Gain2/1

== system ship_induction_motor_propulsion_extended_linear/Controller/Frequency adjustment ==
  Flux_dr_est : Inport
  i_qs : Inport  Port=2
  Gain2 : Gain  Gain=r_r_ind*L_M_ind/(L_M_ind+L_lr_ind)
  Product2 : Product  Inputs=*/
  Saturation : Saturate  UpperLimit=inf  LowerLimit=1e-5
  d_w_e : Outport
  wires:
  i_qs/1 -> Product2/1
  Product2/1 -> Gain2/1
  Saturation/1 -> Product2/2
  Gain2/1 -> d_w_e/1
  Flux_dr_est/1 -> Saturation/1

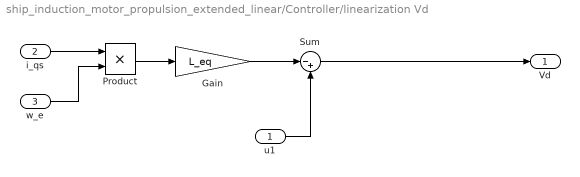
== system ship_induction_motor_propulsion_extended_linear/Controller/linearization Vd ==
  u1 : Inport
  i_qs : Inport  Port=2
  w_e : Inport  Port=3
  Gain : Gain  Gain=L_eq
  Product : Product
  Sum : Sum  Inputs=|-+
  Vd : Outport
  wires:
  u1/1 -> Sum/2
  i_qs/1 -> Product/1
  w_e/1 -> Product/2
  Product/1 -> Gain/1
  Sum/1 -> Vd/1
  Gain/1 -> Sum/1

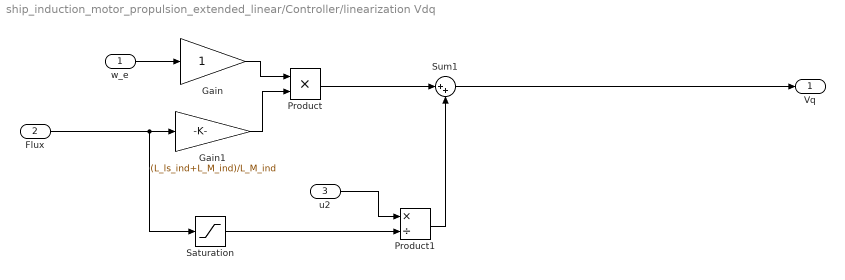
== system ship_induction_motor_propulsion_extended_linear/Controller/linearization Vdq ==
  w_e : Inport
  Flux : Inport  Port=2
  u2 : Inport  Port=3
  Gain : Gain
  Gain1 : Gain  Gain=(L_ls_ind+L_M_ind)/L_M_ind
  Product : Product
  Product1 : Product  Inputs=*/
  Saturation : Saturate  UpperLimit=inf  LowerLimit=1e-5
  Sum1 : Sum  Inputs=|++
  Vq : Outport
  wires:
  Gain1/1 -> Product/2
  Flux/1 -> Saturation/1, Gain1/1
  u2/1 -> Product1/1
  Sum1/1 -> Vq/1
  Product/1 -> Sum1/1
  Product1/1 -> Sum1/2
  Saturation/1 -> Product1/2
  w_e/1 -> Gain/1
  Gain/1 -> Product/1

== matlab function ship_induction_motor_propulsion_extended_linear/Watermarking/Noise Generation ==
  data: prs_noise output; hashing_noise output; x_noise output; x input; N parameter; F parameter; Ts parameter; Seed parameter
function [prs_noise,hashing_noise,   x_noise]= fcn(x,N, F, Ts, Seed)

Ts_noise = 1/F;
SensorNoise = 1;
NoiseMagnitude = N;

if ~SensorNoise 
    x_noise = x;
    hashing_noise = zeros(length(x),1);
    return;
end


persistent t noise ms register uniqueLength stages weights HashR x_noise_1;
%% Initialisation
if isempty(t) 
    % Random number algorithm intitialization 
%     stages = 5;
%     uniqueLength = 5;
%     weights=[1, 1, 2, 1, 2];

%     stages = 3;
%     uniqueLength = 5;
%     weights=[1,1,2,0,2];

%     stages = 3;
%     uniqueLength = 7;
%     weights=[0,2,2,1,2,2,2];

    %% PR M-sequence parameters and generation
    % Initialization of Pseudo Random M-sequence calculation
    stag = 31;
    uniqueLen = 4;
    % Running the search for the primitive polynom weights
    %poly_weights = mseqSearchSiemens(stages, uniqueLen, 1);
    poly_weights =[0     0     2     9];
    period=stag^uniqueLen-1;
    register1=ones(uniqueLen,1);

    mseqence=zeros(1000,1);
    HashR =zeros(1000,1);
    reg_start = register1;

    %% M-sequence calculation
    for i=1:1000
      % calculating next sequence state with modulo stages arithmetic
      % register
      mseqence(i)=rem(poly_weights*register1+stag,stag);
      HashR(i) = (mseqence(i)- floor(stag/2))/(stag-1);
      % updating the register
      register1=[mseqence(i); register1(1:uniqueLen-1)];

      if register1 == reg_start
        % If register is the same as on the beggingin the period polynom is not
        % primitive
        break 
      end
    end
    
    
    t=0;
    noise = zeros(length(x),1);   
    stages = 7;
    uniqueLength = 5;
    weights=[1,3,1,4,3];
    ms = 0;

    
    register = round(rem(ones(1,uniqueLength)*Seed,stages));
    
    x_noise_1 = 0;
else
    t=t+1;
    ms=rem(register*weights'+stages,stages);
    register=[ms, register(:,1:uniqueLength-1)];
    noise = NoiseMagnitude'.* (ms - floor(stages/2))/(stages-1); % eg. 5 stages 0 1 2 3 4 5 -> -2 -1 0 1 2
        
end

x_noise = x + noise;
hashing_noise = NoiseMagnitude'*HashPM1(x_noise_1,HashR);
prs_noise = noise;
x_noise =x_noise+hashing_noise;
x_noise_1 = x + noise;
end

function b = bipolar(a)
b = 2*a-1;
end


%% Simplified Hashing function
% The upper one did not work properly so I created this simplified one, I
% did not want to touch your code :)
function y = HashPM1(in, hash_dict)
% dictionary length
dict_len=length(hash_dict);
y = zeros(size(in));
% Simple index search 
% Signal bounded on [-10,10]
idx_dict = mod(round((in+1)/2 * dict_len),dict_len)+1;
y = hash_dict(idx_dict);
end

== matlab function ship_induction_motor_propulsion_extended_linear/Watermarking2/Noise Generation ==
  data: prs_noise output; hashing_noise output; x_noise output; x input; N parameter; F parameter; Ts parameter; Seed parameter
function [prs_noise,hashing_noise,   x_noise]= fcn(x,N, F, Ts, Seed)

Ts_noise = 1/F;
SensorNoise = 1;
NoiseMagnitude = N;

if ~SensorNoise 
    x_noise = x;
    hashing_noise = zeros(length(x),1);
    return;
end


persistent t noise ms register uniqueLength stages weights HashR x_noise_1;
%% Initialisation
if isempty(t) 
    % Random number algorithm intitialization 
%     stages = 5;
%     uniqueLength = 5;
%     weights=[1, 1, 2, 1, 2];

%     stages = 3;
%     uniqueLength = 5;
%     weights=[1,1,2,0,2];

%     stages = 3;
%     uniqueLength = 7;
%     weights=[0,2,2,1,2,2,2];

    %% PR M-sequence parameters and generation
    % Initialization of Pseudo Random M-sequence calculation
    stag = 31;
    uniqueLen = 4;
    % Running the search for the primitive polynom weights
    %poly_weights = mseqSearchSiemens(stages, uniqueLen, 1);
    poly_weights =[0     0     2     9];
    period=stag^uniqueLen-1;
    register1=ones(uniqueLen,1);

    mseqence=zeros(1000,1);
    HashR =zeros(1000,1);
    reg_start = register1;

    %% M-sequence calculation
    for i=1:1000
      % calculating next sequence state with modulo stages arithmetic
      % register
      mseqence(i)=rem(poly_weights*register1+stag,stag);
      HashR(i) = (mseqence(i)- floor(stag/2))/(stag-1);
      % updating the register
      register1=[mseqence(i); register1(1:uniqueLen-1)];

      if register1 == reg_start
        % If register is the same as on the beggingin the period polynom is not
        % primitive
        break 
      end
    end
    
    
    t=0;
    noise = zeros(length(x),1);   
    stages = 7;
    uniqueLength = 5;
    weights=[1,3,1,4,3];
    ms = 0;

    
    register = round(rem(ones(1,uniqueLength)*Seed,stages));
    
    x_noise_1 = 0;
else
    t=t+1;
    ms=rem(register*weights'+stages,stages);
    register=[ms, register(:,1:uniqueLength-1)];
    noise = NoiseMagnitude'.* (ms - floor(stages/2))/(stages-1); % eg. 5 stages 0 1 2 3 4 5 -> -2 -1 0 1 2
        
end

x_noise = x + noise;
hashing_noise = NoiseMagnitude'*HashPM1(x_noise_1,HashR);
prs_noise = noise;
x_noise =x_noise+hashing_noise;
x_noise_1 = x + noise;
end

function b = bipolar(a)
b = 2*a-1;
end


%% Simplified Hashing function
% The upper one did not work properly so I created this simplified one, I
% did not want to touch your code :)
function y = HashPM1(in, hash_dict)
% dictionary length
dict_len=length(hash_dict);
y = zeros(size(in));
% Simple index search 
% Signal bounded on [-10,10]
idx_dict = mod(round((in+1)/2 * dict_len),dict_len)+1;
y = hash_dict(idx_dict);
end

== matlab function ship_induction_motor_propulsion_extended_linear/Watermarking1/Noise Generation ==
  data: prs_noise output; hashing_noise output; x_noise output; x input; N parameter; F parameter; Ts parameter; Seed parameter
function [prs_noise,hashing_noise,   x_noise]= fcn(x,N, F, Ts, Seed)

Ts_noise = 1/F;
SensorNoise = 1;
NoiseMagnitude = N;

if ~SensorNoise 
    x_noise = x;
    hashing_noise = zeros(length(x),1);
    return;
end


persistent t noise ms register uniqueLength stages weights HashR x_noise_1;
%% Initialisation
if isempty(t) 
    % Random number algorithm intitialization 
%     stages = 5;
%     uniqueLength = 5;
%     weights=[1, 1, 2, 1, 2];

%     stages = 3;
%     uniqueLength = 5;
%     weights=[1,1,2,0,2];

%     stages = 3;
%     uniqueLength = 7;
%     weights=[0,2,2,1,2,2,2];

    %% PR M-sequence parameters and generation
    % Initialization of Pseudo Random M-sequence calculation
    stag = 31;
    uniqueLen = 4;
    % Running the search for the primitive polynom weights
    %poly_weights = mseqSearchSiemens(stages, uniqueLen, 1);
    poly_weights =[0     0     2     9];
    period=stag^uniqueLen-1;
    register1=ones(uniqueLen,1);

    mseqence=zeros(1000,1);
    HashR =zeros(1000,1);
    reg_start = register1;

    %% M-sequence calculation
    for i=1:1000
      % calculating next sequence state with modulo stages arithmetic
      % register
      mseqence(i)=rem(poly_weights*register1+stag,stag);
      HashR(i) = (mseqence(i)- floor(stag/2))/(stag-1);
      % updating the register
      register1=[mseqence(i); register1(1:uniqueLen-1)];

      if register1 == reg_start
        % If register is the same as on the beggingin the period polynom is not
        % primitive
        break 
      end
    end
    
    
    t=0;
    noise = zeros(length(x),1);   
    stages = 7;
    uniqueLength = 5;
    weights=[1,3,1,4,3];
    ms = 0;

    
    register = round(rem(ones(1,uniqueLength)*Seed,stages));
    
    x_noise_1 = 0;
else
    t=t+1;
    ms=rem(register*weights'+stages,stages);
    register=[ms, register(:,1:uniqueLength-1)];
    noise = NoiseMagnitude'.* (ms - floor(stages/2))/(stages-1); % eg. 5 stages 0 1 2 3 4 5 -> -2 -1 0 1 2
        
end

x_noise = x + noise;
hashing_noise = NoiseMagnitude'*HashPM1(x_noise_1,HashR);
prs_noise = noise;
x_noise =x_noise+hashing_noise;
x_noise_1 = x + noise;
end

function b = bipolar(a)
b = 2*a-1;
end


%% Simplified Hashing function
% The upper one did not work properly so I created this simplified one, I
% did not want to touch your code :)
function y = HashPM1(in, hash_dict)
% dictionary length
dict_len=length(hash_dict);
y = zeros(size(in));
% Simple index search 
% Signal bounded on [-10,10]
idx_dict = mod(round((in+1)/2 * dict_len),dict_len)+1;
y = hash_dict(idx_dict);
end

== matlab function ship_induction_motor_propulsion_extended_linear/Watermarking test1/Noise Generation1 ==
  data: x_recovered output; x input; N parameter; F parameter; Ts parameter; Seed parameter
function x_recovered  = fcn(x,N, F, Ts, Seed)

Ts_noise = 1/F;
SensorNoise = 1;
NoiseMagnitude = N;

if ~SensorNoise 
    x_noise = x;
    hashing_noise = zeros(length(x),1);
    return;
end


persistent t prs_noise ms register uniqueLength stages weights HashR x_rec_1 prs_noise_1 x_rec;
%% Initialisation
if isempty(t) 
    % Random number algorithm intitialization 
%     stages = 5;
%     uniqueLength = 5;
%     weights=[1, 1, 2, 1, 2];

%     stages = 3;
%     uniqueLength = 5;
%     weights=[1,1,2,0,2];

%     stages = 3;
%     uniqueLength = 7;
%     weights=[0,2,2,1,2,2,2];

    %% PR M-sequence parameters and generation
    % Initialization of Pseudo Random M-sequence calculation
    stag = 31;
    uniqueLen = 4;
    % Running the search for the primitive polynom weights
    %poly_weights = mseqSearchSiemens(stages, uniqueLen, 1);
    poly_weights =[0     0     2     9];
    period=stag^uniqueLen-1;
    register1=ones(uniqueLen,1);

    mseqence=zeros(1000,1);
    HashR =zeros(1000,1);
    reg_start = register1;
    
    %% M-sequence calculation
    for i=1:1000
      % calculating next sequence state with modulo stages arithmetic
      % register
      mseqence(i)=rem(poly_weights*register1+stag,stag);
      HashR(i) = (mseqence(i)- floor(stag/2))/(stag-1);
      % updating the register
      register1=[mseqence(i); register1(1:uniqueLen-1)];

      if register1 == reg_start
        % If register is the same as on the beggingin the period polynom is not
        % primitive
        break 
      end
    end
    
    
    t=0;
    prs_noise = zeros(length(x),1);   
    stages = 7;
    uniqueLength = 5;
    weights=[1,3,1,4,3];
    ms = 0;
    
    register = round(rem(ones(1,uniqueLength)*Seed,stages));
    
    x_rec = 0;
    x_rec_1 = 0;
    
else
    t=t+1;
        
    prs_noise_1 = prs_noise;
    ms=rem(register*weights'+stages,stages);
    register=[ms, register(:,1:uniqueLength-1)];
    prs_noise = NoiseMagnitude'.* (ms - floor(stages/2))/(stages-1); % eg. 5 stages 0 1 2 3 4 5 -> -2 -1 0 1 2
    x_rec = x - prs_noise - NoiseMagnitude'*HashPM1(x_rec_1 + prs_noise_1, HashR);
    

end
x_recovered= x_rec;

x_rec_1 = x_rec;
end

function b = bipolar(a)
b = 2*a-1;
end


%% Simplified Hashing function
% The upper one did not work properly so I created this simplified one, I
% did not want to touch your code :)
function y = HashPM1(in, hash_dict)
% dictionary length
dict_len=length(hash_dict);
y = zeros(size(in));
% Simple index search 
% Signal bounded on [-10,10]
idx_dict = mod(round((in+1)/2 * dict_len),dict_len)+1;
y = hash_dict(idx_dict);
end

== matlab function ship_induction_motor_propulsion_extended_linear/Watermarking test1/Test Function ==
  data: y input; gk_chi output; gk_chi_av output; y_attack input; gk_sub output
function [gk_chi,gk_chi_av, gk_sub] = fcn(y,y_attack)


persistent Y Y_attack Variance GK n

wind =20;
if isempty(Y)
    n = 0;
    Y = zeros(wind,1);
    Y_attack = zeros(wind,1);
    Variance = 1e-7;
    GK = zeros(wind,1);
else
    if(n > 2)
        % simple system dynamics compensation
        dY = Y(1)-Y(2);
        %dY = 0;
    else
        dY = 0;
    end
    Y = [y; Y(1:end-1)];
    Y_attack = [y_attack+dY; Y_attack(1:end-1,:)];
    n=n+1;
end

% mean = sum(Y_attack)/wind;
% stdev = 1/wind*sqrt(sum((Y_attack-wind).^2));
% gk = stdev;
gk_chi = log10(sum((Y-Y_attack).*Variance^-1.*(Y-Y_attack)));
gk_chi_av = abs(sum(GK))/wind;
GK = [gk_chi; GK(1:end-1)];
gk_sub = Y(1,:)-Y_attack(2,:);

== matlab function ship_induction_motor_propulsion_extended_linear/Watermarking test/Test Function ==
  data: y input; gk_chi output; gk_chi_av output; y_attack input; gk_sub output
function [gk_chi,gk_chi_av, gk_sub] = fcn(y,y_attack)


persistent Y Y_attack Variance GK n

wind =10;
if isempty(Y)
    n = 0;
    Y = zeros(wind,1);
    Y_attack = zeros(wind,1);
    Variance = 1e-7;
    GK = zeros(wind,1);
else
    if(n > 2)
        % simple system dynamics compensation
        dY = Y(1)-Y(2);
        %dY = 0;
    else
        dY = 0;
    end
    Y = [y; Y(1:end-1)];
    Y_attack = [y_attack+dY; Y_attack(1:end-1,:)];
    n=n+1;
end

% mean = sum(Y_attack)/wind;
% stdev = 1/wind*sqrt(sum((Y_attack-wind).^2));
% gk = stdev;
gk_chi = log10(sum((Y-Y_attack).*Variance^-1.*(Y-Y_attack)));
gk_chi_av = abs(sum(GK))/wind;
GK = [gk_chi; GK(1:end-1)];
gk_sub = Y(1,:)-Y_attack(2,:);

== matlab function ship_induction_motor_propulsion_extended_linear/Watermarking test/Noise Generation1 ==
  data: x_recovered output; x input; N parameter; F parameter; Ts parameter; Seed parameter
function x_recovered  = fcn(x,N, F, Ts, Seed)

Ts_noise = 1/F;
SensorNoise = 1;
NoiseMagnitude = N;

if ~SensorNoise 
    x_noise = x;
    hashing_noise = zeros(length(x),1);
    return;
end


persistent t prs_noise ms register uniqueLength stages weights HashR x_rec_1 prs_noise_1 x_rec;
%% Initialisation
if isempty(t) 
    % Random number algorithm intitialization 
%     stages = 5;
%     uniqueLength = 5;
%     weights=[1, 1, 2, 1, 2];

%     stages = 3;
%     uniqueLength = 5;
%     weights=[1,1,2,0,2];

%     stages = 3;
%     uniqueLength = 7;
%     weights=[0,2,2,1,2,2,2];

    %% PR M-sequence parameters and generation
    % Initialization of Pseudo Random M-sequence calculation
    stag = 31;
    uniqueLen = 4;
    % Running the search for the primitive polynom weights
    %poly_weights = mseqSearchSiemens(stages, uniqueLen, 1);
    poly_weights =[0     0     2     9];
    period=stag^uniqueLen-1;
    register1=ones(uniqueLen,1);

    mseqence=zeros(1000,1);
    HashR =zeros(1000,1);
    reg_start = register1;
    
    %% M-sequence calculation
    for i=1:1000
      % calculating next sequence state with modulo stages arithmetic
      % register
      mseqence(i)=rem(poly_weights*register1+stag,stag);
      HashR(i) = (mseqence(i)- floor(stag/2))/(stag-1);
      % updating the register
      register1=[mseqence(i); register1(1:uniqueLen-1)];

      if register1 == reg_start
        % If register is the same as on the beggingin the period polynom is not
        % primitive
        break 
      end
    end
    
    
    t=0;
    prs_noise = zeros(length(x),1);   
    stages = 7;
    uniqueLength = 5;
    weights=[1,3,1,4,3];
    ms = 0;
    
    register = round(rem(ones(1,uniqueLength)*Seed,stages));
    
    x_rec = 0;
    x_rec_1 = 0;
    
else
    t=t+1;
        
    prs_noise_1 = prs_noise;
    ms=rem(register*weights'+stages,stages);
    register=[ms, register(:,1:uniqueLength-1)];
    prs_noise = NoiseMagnitude'.* (ms - floor(stages/2))/(stages-1); % eg. 5 stages 0 1 2 3 4 5 -> -2 -1 0 1 2
    x_rec = x - prs_noise - NoiseMagnitude'*HashPM1(x_rec_1 + prs_noise_1, HashR);
    

end
x_recovered= x_rec;

x_rec_1 = x_rec;
end

function b = bipolar(a)
b = 2*a-1;
end


%% Simplified Hashing function
% The upper one did not work properly so I created this simplified one, I
% did not want to touch your code :)
function y = HashPM1(in, hash_dict)
% dictionary length
dict_len=length(hash_dict);
y = zeros(size(in));
% Simple index search 
% Signal bounded on [-10,10]
idx_dict = mod(round((in+1)/2 * dict_len),dict_len)+1;
y = hash_dict(idx_dict);
end

== matlab function ship_induction_motor_propulsion_extended_linear/Watermarking test2/Noise Generation1 ==
  data: x_recovered output; x input; N parameter; F parameter; Ts parameter; Seed parameter
function x_recovered  = fcn(x,N, F, Ts, Seed)

Ts_noise = 1/F;
SensorNoise = 1;
NoiseMagnitude = N;

if ~SensorNoise 
    x_noise = x;
    hashing_noise = zeros(length(x),1);
    return;
end


persistent t prs_noise ms register uniqueLength stages weights HashR x_rec_1 prs_noise_1 x_rec;
%% Initialisation
if isempty(t) 
    % Random number algorithm intitialization 
%     stages = 5;
%     uniqueLength = 5;
%     weights=[1, 1, 2, 1, 2];

%     stages = 3;
%     uniqueLength = 5;
%     weights=[1,1,2,0,2];

%     stages = 3;
%     uniqueLength = 7;
%     weights=[0,2,2,1,2,2,2];

    %% PR M-sequence parameters and generation
    % Initialization of Pseudo Random M-sequence calculation
    stag = 31;
    uniqueLen = 4;
    % Running the search for the primitive polynom weights
    %poly_weights = mseqSearchSiemens(stages, uniqueLen, 1);
    poly_weights =[0     0     2     9];
    period=stag^uniqueLen-1;
    register1=ones(uniqueLen,1);

    mseqence=zeros(1000,1);
    HashR =zeros(1000,1);
    reg_start = register1;
    
    %% M-sequence calculation
    for i=1:1000
      % calculating next sequence state with modulo stages arithmetic
      % register
      mseqence(i)=rem(poly_weights*register1+stag,stag);
      HashR(i) = (mseqence(i)- floor(stag/2))/(stag-1);
      % updating the register
      register1=[mseqence(i); register1(1:uniqueLen-1)];

      if register1 == reg_start
        % If register is the same as on the beggingin the period polynom is not
        % primitive
        break 
      end
    end
    
    
    t=0;
    prs_noise = zeros(length(x),1);   
    stages = 7;
    uniqueLength = 5;
    weights=[1,3,1,4,3];
    ms = 0;
    
    register = round(rem(ones(1,uniqueLength)*Seed,stages));
    
    x_rec = 0;
    x_rec_1 = 0;
    
else
    t=t+1;
        
    prs_noise_1 = prs_noise;
    ms=rem(register*weights'+stages,stages);
    register=[ms, register(:,1:uniqueLength-1)];
    prs_noise = NoiseMagnitude'.* (ms - floor(stages/2))/(stages-1); % eg. 5 stages 0 1 2 3 4 5 -> -2 -1 0 1 2
    x_rec = x - prs_noise - NoiseMagnitude'*HashPM1(x_rec_1 + prs_noise_1, HashR);
    

end
x_recovered= x_rec;

x_rec_1 = x_rec;
end

function b = bipolar(a)
b = 2*a-1;
end


%% Simplified Hashing function
% The upper one did not work properly so I created this simplified one, I
% did not want to touch your code :)
function y = HashPM1(in, hash_dict)
% dictionary length
dict_len=length(hash_dict);
y = zeros(size(in));
% Simple index search 
% Signal bounded on [-10,10]
idx_dict = mod(round((in+1)/2 * dict_len),dict_len)+1;
y = hash_dict(idx_dict);
end

== matlab function ship_induction_motor_propulsion_extended_linear/Watermarking test2/Test Function ==
  data: y input; gk_chi output; gk_chi_av output; y_attack input; gk_sub output
function [gk_chi,gk_chi_av, gk_sub] = fcn(y,y_attack)


persistent Y Y_attack Variance GK n

wind =20;
if isempty(Y)
    n = 0;
    Y = zeros(wind,1);
    Y_attack = zeros(wind,1);
    Variance = 1e-7;
    GK = zeros(wind,1);
else
    if(n > 2)
        % simple system dynamics compensation
        dY = Y(1)-Y(2);
        %dY = 0;
    else
        dY = 0;
    end
    Y = [y; Y(1:end-1)];
    Y_attack = [y_attack+dY; Y_attack(1:end-1,:)];
    n=n+1;
end

% mean = sum(Y_attack)/wind;
% stdev = 1/wind*sqrt(sum((Y_attack-wind).^2));
% gk = stdev;
gk_chi = log10(sum((Y-Y_attack).*Variance^-1.*(Y-Y_attack)));
gk_chi_av = abs(sum(GK))/wind;
GK = [gk_chi; GK(1:end-1)];
gk_sub = Y(1,:)-Y_attack(2,:);
